simulink model "euler_transform_folded"  (R2018b)
settings: Solver=FixedStepAuto  StartTime=0.0  StopTime=100000  FixedStep=1  RelTol=1e-3
undefined symbols (not defined in the file or in its folder): nIters, phiVals, psiVals, selData, thetaVals, uIn
libraries: cordic_rotation_mode x2, simulink x1, hdlsllib x1
settings Model: Creator=jimjoy  LastModifiedBy=tbryan

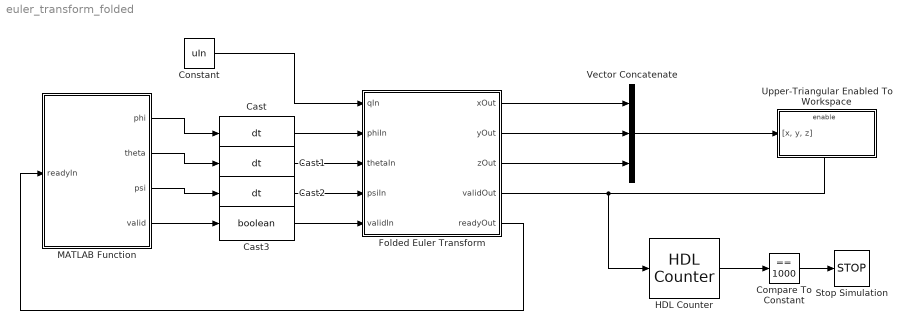
== system euler_transform_folded ==
  Cast : DataTypeConversion  OutDataTypeStr=dt
  Cast1 : DataTypeConversion  OutDataTypeStr=dt
  Cast2 : DataTypeConversion  OutDataTypeStr=dt
  Cast3 : DataTypeConversion  OutDataTypeStr=boolean
  Compare To Constant : simulink/Logic and Bit Operations/Compare To Constant  relop===  const=1000  OutDataTypeStr=boolean
  Constant : Constant  Value=uIn
  Folded Euler Transform : Subsystem
  HDL Counter : hdlsllib/Sources/HDL Counter  CountType=Free running  CountInit=0  CountStep=1  CountMax=25  CountFromType=Initial value  CountFrom=0  CountResetPort=off  CountLoadPort=off  CountEnbPort=on  CountDirPort=off  CountDataType=Unsigned  CountWordLen=16  CountFracLen=0  CountSampTime=1
      settings: SourceProductName=Simulink
  MATLAB Function : MATLAB Function  TreatAsAtomicUnit=on  mask{phiVals=phiVals, thetaVals=thetaVals, psiVals=psiVals, selData=selData}
      mask prompts: phiVals "phi"; thetaVals "theta"; psiVals "psi"; selData "Select data"
  Stop Simulation : Stop
  Upper-Triangular Enabled To Workspace : Subsystem  mask{VariableName=uOut}
      mask prompts: VariableName "Variable name:"
      mask init:
      | obj = get_param(gcbh,'object');
      | twObj = get_param([gcb '/To Workspace'],'object');
      | twObj.VariableName = obj.VariableName;
      mask Display: disp(VariableName);
  Vector Concatenate : Concatenate  NumInputs=3
  wires:
  MATLAB Function/1(phi) -> Cast/1
  MATLAB Function/2(theta) -> Cast1/1
  MATLAB Function/3(psi) -> Cast2/1
  MATLAB Function/4(valid) -> Cast3/1
  Folded Euler Transform/5(readyOut) -> MATLAB Function/1(readyIn)
  Folded Euler Transform/1(xOut) -> Vector Concatenate/1
  Folded Euler Transform/2(yOut) -> Vector Concatenate/2
  Folded Euler Transform/3(zOut) -> Vector Concatenate/3
  Folded Euler Transform/4(validOut) -> Upper-Triangular Enabled To Workspace/Enable, HDL Counter/1
  Constant/1 -> Folded Euler Transform/1(qIn)
  Cast/1 -> Folded Euler Transform/2(phiIn)
  Cast1/1 -> Folded Euler Transform/3(thetaIn)
  Cast2/1 -> Folded Euler Transform/4(psiIn)
  Cast3/1 -> Folded Euler Transform/5(validIn)
  Vector Concatenate/1 -> Upper-Triangular Enabled To Workspace/1("[x, y, z]")
  HDL Counter/1 -> Compare To Constant/1
  Compare To Constant/1 -> Stop Simulation/1

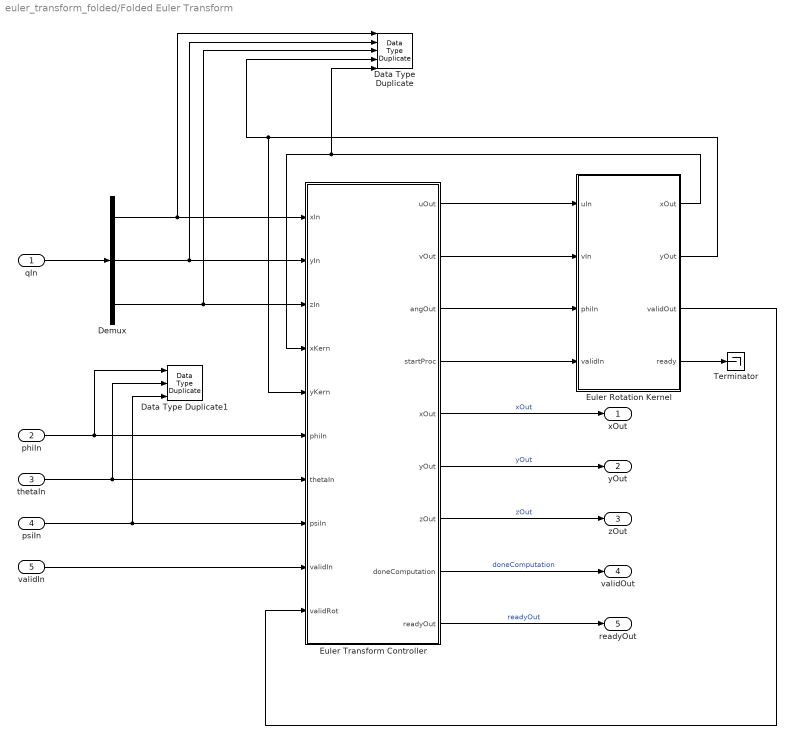
== system euler_transform_folded/Folded Euler Transform ==
  qIn : Inport
  phiIn : Inport  Port=2
  thetaIn : Inport  Port=3
  psiIn : Inport  Port=4
  validIn : Inport  Port=5
  Data Type Duplicate : DataTypeDuplicate  NumInputPorts=5
  Data Type Duplicate1 : DataTypeDuplicate  NumInputPorts=3
  Demux : Demux  Outputs=3
  Euler Rotation Kernel : Subsystem
  Euler Transform Controller : MATLAB Function  TreatAsAtomicUnit=on
  Terminator : Terminator
  xOut : Outport  PortDimensions=1
  yOut : Outport  Port=2  PortDimensions=1
  zOut : Outport  Port=3  PortDimensions=1
  validOut : Outport  Port=4  PortDimensions=1
  readyOut : Outport  Port=5
  wires:
  qIn/1 -> Demux/1
  Demux/1 -> Data Type Duplicate/1, Euler Transform Controller/1(xIn)
  Demux/2 -> Data Type Duplicate/2, Euler Transform Controller/2(yIn)
  Demux/3 -> Data Type Duplicate/3, Euler Transform Controller/3(zIn)
  phiIn/1 -> Data Type Duplicate1/1, Euler Transform Controller/6(phiIn)
  thetaIn/1 -> Data Type Duplicate1/2, Euler Transform Controller/7(thetaIn)
  psiIn/1 -> Data Type Duplicate1/3, Euler Transform Controller/8(psiIn)
  validIn/1 -> Euler Transform Controller/9(validIn)
  Euler Rotation Kernel/3(validOut) -> Euler Transform Controller/10(validRot)
  Euler Rotation Kernel/1(xOut) -> Data Type Duplicate/5, Euler Transform Controller/4(xKern)
  Euler Rotation Kernel/2(yOut) -> Data Type Duplicate/4, Euler Transform Controller/5(yKern)
  Euler Transform Controller/1(uOut) -> Euler Rotation Kernel/1(uIn)
  Euler Transform Controller/2(vOut) -> Euler Rotation Kernel/2(vIn)
  Euler Transform Controller/3(angOut) -> Euler Rotation Kernel/3(phiIn)
  Euler Transform Controller/4(startProc) -> Euler Rotation Kernel/4(validIn)
  Euler Transform Controller/8(doneComputation) -> validOut/1  "doneComputation"
  Euler Transform Controller/5(xOut) -> xOut/1  "xOut"
  Euler Transform Controller/6(yOut) -> yOut/1  "yOut"
  Euler Transform Controller/7(zOut) -> zOut/1  "zOut"
  Euler Transform Controller/9(readyOut) -> readyOut/1  "readyOut"
  Euler Rotation Kernel/4(ready) -> Terminator/1

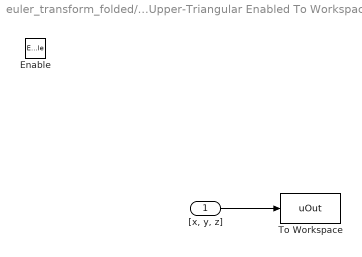
== system euler_transform_folded/Upper-Triangular Enabled To Workspace ==
  "[x, y, z]" : Inport
  Enable : EnablePort
  To Workspace : ToWorkspace  VariableName=uOut  SampleTime=-1
  wires:
  "[x, y, z]"/1 -> To Workspace/1

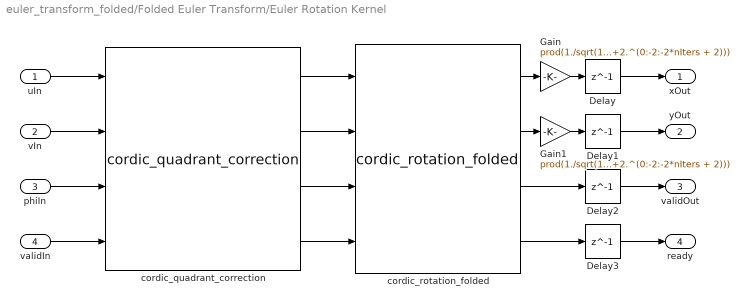
== system euler_transform_folded/Folded Euler Transform/Euler Rotation Kernel ==
  uIn : Inport
  vIn : Inport  Port=2
  phiIn : Inport  Port=3
  validIn : Inport  Port=4
  Delay{,1..3} (4 alike) : Delay  DelayLength=1
  Gain : Gain  Gain=prod(1./sqrt(1+2.^(0:-2:-2*nIters + 2)))  OutDataTypeStr=Inherit: Same as input
  Gain1 : Gain  Gain=prod(1./sqrt(1+2.^(0:-2:-2*nIters + 2)))  OutDataTypeStr=Inherit: Same as input
  cordic_quadrant_correction : cordic_rotation_mode/cordic_quadrant_correction  SystemSampleTime=-1
  cordic_rotation_folded : cordic_rotation_mode/cordic_rotation_folded  nIters=nIters
  xOut : Outport
  yOut : Outport  Port=2
  validOut : Outport  Port=3
  ready : Outport  Port=4  PortDimensions=1
  wires:
  uIn/1 -> cordic_quadrant_correction/1
  vIn/1 -> cordic_quadrant_correction/2
  phiIn/1 -> cordic_quadrant_correction/3
  validIn/1 -> cordic_quadrant_correction/4
  cordic_quadrant_correction/1 -> cordic_rotation_folded/1
  cordic_quadrant_correction/2 -> cordic_rotation_folded/2
  cordic_quadrant_correction/3 -> cordic_rotation_folded/3
  cordic_quadrant_correction/4 -> cordic_rotation_folded/4
  Gain1/1 -> Delay1/1
  cordic_rotation_folded/4 -> Delay3/1
  cordic_rotation_folded/3 -> Delay2/1
  Gain/1 -> Delay/1
  cordic_rotation_folded/2 -> Gain1/1
  cordic_rotation_folded/1 -> Gain/1
  Delay/1 -> xOut/1
  Delay1/1 -> yOut/1
  Delay2/1 -> validOut/1
  Delay3/1 -> ready/1

== matlab function euler_transform_folded/MATLAB Function ==
  settings: fimath=hdlfimath
  data: phiVals parameter; thetaVals parameter; psiVals parameter; phi output; theta output; psi output; valid output; selData parameter; readyIn input
function [phi, theta, psi, valid] = generateData(phiVals, thetaVals, psiVals, selData, readyIn)
%#codegen

persistent phiReg thetaReg psiReg validReg ii

if isempty(phiReg)
    phiReg = cast(0,'like',phiVals);
    thetaReg = cast(0,'like',thetaVals);
    psiReg = cast(0,'like',psiVals);
    validReg = false;
    ii = 1;
end

phi = phiReg(:);
theta = thetaReg(:);
psi = psiReg(:);
valid = validReg;

validReg(:) = false;
if readyIn
    switch selData
        case 0
            phiReg(:) = phiVals(ii);
            thetaReg(:) = thetaVals(1);
            psiReg(:) = psiVals(1);
            ll = length(phiVals);
        case 1
            phiReg(:) = phiVals(1);
            thetaReg(:) = thetaVals(ii);
            psiReg(:) = psiVals(1);
            ll = length(thetaVals);
        case 2
            phiReg(:) = phiVals(1);
            thetaReg(:) = thetaVals(1);
            psiReg(:) = psiVals(ii);
            ll = length(psiVals);
    end
    if ii < ll
        ii = ii + 1;
    else
        ii = 1;
    end
    validReg(:) = true;
end

== matlab function euler_transform_folded/Folded Euler Transform/Euler Transform Controller ==
  settings: fimath=hdlfimath
  data: xIn input; uOut output size=[1 1]; yIn input; zIn input; xKern input; yKern input; phiIn input; thetaIn input; psiIn input; validIn input; validRot input; vOut output size=[1 1]; angOut output size=[1 1]; startProc output size=[1]; xOut output; yOut output; zOut output; doneComputation output; readyOut output size=1
function [uOut, vOut, angOut, startProc, xOut, yOut, zOut, doneComputation, readyOut]  = ...
        eulerTransformController(xIn, yIn, zIn, xKern, yKern, phiIn, thetaIn, psiIn, validIn, validRot)
    
    % Copyright 2018 The MathWorks, Inc.
    
    persistent xReg yReg zReg xBuff yBuff zBuff
    persistent phiReg thetaReg psiReg
    persistent phiBuff thetaBuff psiBuff buffFull
    persistent readyReg procReg doneReg
    persistent uReg vReg angReg
    persistent state stepNum
    
    % Get the types table
    T = getTypesTable(xIn, yIn, zIn, phiIn, thetaIn, psiIn);
    
    % Define states for control logic for Euler Rotation Kernel
    numKernelStates = coder.const(3);
    kernelStateWordLength = nextpow2(numKernelStates);
    kernelStateNumericType = numerictype(0,kernelStateWordLength,0);
    idle = fi(0, kernelStateNumericType);
    processing = fi(1, kernelStateNumericType);
    setOutputRegisters = fi(3,kernelStateNumericType);
    
    % Initialize persistent variables
    if isempty(xReg)
        xReg = cast(0,'like',T.x);
        yReg = cast(0,'like',T.y);
        zReg = cast(0,'like',T.z);
        xBuff = cast(0,'like',T.x);
        yBuff = cast(0,'like',T.y);
        zBuff = cast(0,'like',T.z);
        phiReg = cast(0,'like',T.phi);
        thetaReg = cast(0,'like',T.theta);
        psiReg = cast(0,'like',T.psi);
        phiBuff = cast(0,'like',T.phi);
        thetaBuff = cast(0,'like',T.theta);
        psiBuff = cast(0,'like',T.psi);
        uReg = cast(0,'like',T.x);
        vReg = cast(0,'like',T.x);
        angReg = cast(0,'like',T.phi);
        readyReg = true;
        procReg = false;
        doneReg = false;
        state = idle;
       	buffFull = false;
        stepNum = fi(0,0,2,0,hdlfimath);
    end
    
    % Assign defaults to outputs for datatyping purposes
    uOut = cast(0,'like',T.x);
    vOut = cast(0,'like',T.y);
    xOut = cast(0,'like',T.x);
    yOut = cast(0,'like',T.y);
    zOut = cast(0,'like',T.z);
    angOut = cast(0,'like',T.phi);
    startProc = cast(false,'like',T.validIn);
    doneComputation = cast(false,'like',T.validIn);
    readyOut = cast(false,'like',T.validIn);
    
    % Define states to buffer data if necessary
    
    % Assign outputs
    uOut(:) = uReg;
    vOut(:) = vReg;
    angOut(:) = angReg;
    startProc(:) = procReg;
    xOut(:) = xReg;
    yOut(:) = yReg;
    zOut(:) = zReg;
    doneComputation(:) = doneReg;
    readyOut(:) = readyReg;
    
    % Read from buffer if there is data there
    phiNext = cast(0,'like',T.phi);
    thetaNext = cast(0,'like', T.theta);
    psiNext = cast(0,'like',T.psi);
    xNext = cast(0,'like',T.x);
    yNext = cast(0,'like',T.y);
    zNext = cast(0,'like',T.z);
    if buffFull
        phiNext(:) = phiBuff;
        thetaNext(:) = thetaBuff;
        psiNext(:) = psiBuff;
        xNext(:) = xBuff;
        yNext(:) = yBuff;
        zNext(:) = zBuff;
    else
        phiNext(:) = phiIn;
        thetaNext(:) = thetaIn;
        psiNext(:) = psiIn;
        xNext(:) = xIn;
        yNext(:) = yIn;
        zNext(:) = zIn;
    end
    
    % Fill the buffer, if necessary
    if validIn && ~(buffFull || readyReg)
       xBuff(:) = xIn;
       yBuff(:) = yIn;
       zBuff(:) = zIn;
       phiBuff(:) = phiIn;
       thetaBuff(:) = thetaIn;
       psiBuff(:) = psiIn;
       buffFull(:) = true;
    else
       xBuff(:) = xBuff;
       yBuff(:) = yBuff;
       zBuff(:) = zBuff;
       phiBuff(:) = phiBuff;
       thetaBuff(:) = thetaBuff;
       psiBuff(:) = psiBuff;
       buffFull(:) = buffFull;
    end
        
    
    % State Update
    switch state
        case idle
            doneReg(:) = false;
            angReg(:) = phiNext;
            xReg(:) = xNext;
            yReg(:) = yNext;
            zReg(:) = zNext;
            uReg(:) = yNext;
            vReg(:) = zNext;
            phiReg(:) = phiNext;
            thetaReg(:) = thetaNext;
            psiReg(:) = psiNext;
            if buffFull || (validIn && readyReg)
                readyReg(:) = false;
                state(:) = processing;
                procReg(:) = true;
            else
                readyReg(:) = true;
                state(:) = idle;
                procReg(:) = false;
            end
            buffFull(:) = false;
        case processing
            procReg(:) = false;
            switch stepNum
                case 0
                    xReg(:) = xReg;
                    yReg(:) = xKern;
                    zReg(:) = yKern;
                case 1
                    xReg(:) = xKern;
                    yReg(:) = yReg;
                    zReg(:) = yKern;
                case 2
                    xReg(:) = xKern;
                    yReg(:) = yKern;
                    zReg(:) = zReg;
                otherwise
                    xReg(:) = xReg;
                    yReg(:) = yReg;
                    zReg(:) = zReg;
            end
            if validRot
                state(:) = setOutputRegisters;
                stepNum(:) = stepNum + 1;
            else
                state(:) = processing;
                stepNum(:) = stepNum;
            end
        case setOutputRegisters
            readyReg(:) = false;
            stepNum(:) = stepNum;
            procReg(:) = true;
            state(:) = processing;
            doneReg(:) = false;
            switch stepNum
                case 1
                    uReg(:) = xReg;
                    vReg(:) = zReg;
                    angReg(:) = -thetaReg;
                case 2
                    uReg(:) = xReg;
                    vReg(:) = yReg;
                    angReg(:) = psiReg;
                otherwise
                    uReg(:) = yReg;
                    vReg(:) = zReg;
                    angReg(:) = phiReg;
                    procReg(:) = false;
                    stepNum(:) = 0;
                    readyReg(:) = true;
                    doneReg(:) = true;
                    state(:) = idle;
            end
        otherwise
            xReg(:) = 0;
            yReg(:) = 0;
            zReg(:) = 0;
            xBuff(:) = 0;
            yBuff(:) = 0;
            zBuff(:) = 0;
            phiReg(:) = 0;
            thetaReg(:) = 0;
            psiReg(:) = 0;
            phiBuff(:) = 0;
            thetaBuff(:) = 0;
            psiBuff(:) = 0;
            uReg(:) = 0;
            vReg(:) = 0;
            angReg(:) = 0;
            readyReg(:) = true;
            procReg(:) = false;
            doneReg(:) = false;
            state(:) = idle;
            stepNum(:) = fi(0,0,2,0,hdlfimath);
    end
    
end

function T = getTypesTable(xIn, yIn, zIn, phiIn, thetaIn, psiIn)
    % Assign the types table for the input data
    if isfi(xIn)
        if isfloat(xIn) || isfloat(yIn) || isfloat(zIn)
            assert(~coder.target('HDL'), 'Floating-Point not supported for this function in HDL Code Generation');
            assert((xIn.DataTypeMode == yIn.DataTypeMode) && (yIn.DataTypeMode == zIn.DataTypeMode),...
                'Floating-Point Simulation Requires that x, y, and z have the same datatype')
            T.x = cast([],'like',x);
        else
            assert(isscaledtype(xIn) && isscaledtype(yIn) && isscaledtype(zIn),...
                'Fixed-Point x, y, and z must be scaled types');
            assert((xIn.WordLength == yIn.WordLength) && (xIn.WordLength == zIn.WordLength),...
                'Fixed-Point x, y, and z must have the same wordlengths');
            assert((xIn.FractionLength == yIn.FractionLength) && (xIn.FractionLength == zIn.FractionLength),...
                'Fixed-Point x, y, and z must have the same fraction length');
            wl = max(8, xIn.WordLength);
            fl = min(wl - 3, xIn.FractionLength);
            T.x = fi([],1,wl, fl);
        end
    elseif isfloat(xIn)
        assert(~coder.target('HDL'), 'Floating-Point not supported for this function in HDL Code Generation');
        assert(strcmp(class(xIn),class(yIn))&& strcmp(class(xIn),class(zIn)),...
            'Floating-Point Simulation Requires that x, y, and z have the same datatype');
        T.x = cast([],'like',xIn);
    else
        error('Datatype of x unsupported');
    end
    T.y = cast([],'like',yIn);
    T.z = cast([],'like',zIn);
    if isfi(phiIn)
        if isfloat(phiIn) || isfloat(thetaIn) || isfloat(psiIn)
            assert(~coder.target('HDL'),'Floating-Point not supported for this function in HDL Code Generation');
        end
        T.phi = cast([],'like',phiIn);
        T.theta = cast([],'like',thetaIn);
        T.psi = cast([],'like',psiIn);
    elseif isfloat(phiIn)
        assert(strcmp(class(phiIn),class(thetaIn)) && strcmp(class(phiIn),class(psiIn)),...
            'Angular inputs must have the same floating point type');
        T.phi = cast([],'like',phiIn);
        T.theta = cast([],'like',thetaIn);
        T.psi = cast([],'like',psiIn);
    end
    T.validIn = cast([],'like',true);
    T.validRot = cast([],'like',true);
    T.kernelReady = cast([],'like',true);  
end
